simulink model "cascaded_with_phase_shifted"  (R2022b)
settings: Solver=ode3  StartTime=0.0  StopTime=0.5  FixedStep=5e-5  RelTol=1e-3
libraries: spsIGBTDiodeLib x8, simulink x4, spsDCVoltageSourceLib x2, spsVoltageMeasurementLib x1, sps_lib x1
settings Model: Creator=gudel  LastModifiedBy=gudel

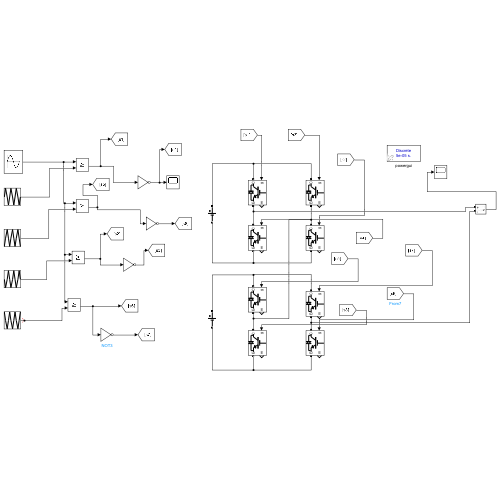
[thumbnail: Simulink's stored preview of the top-level diagram]
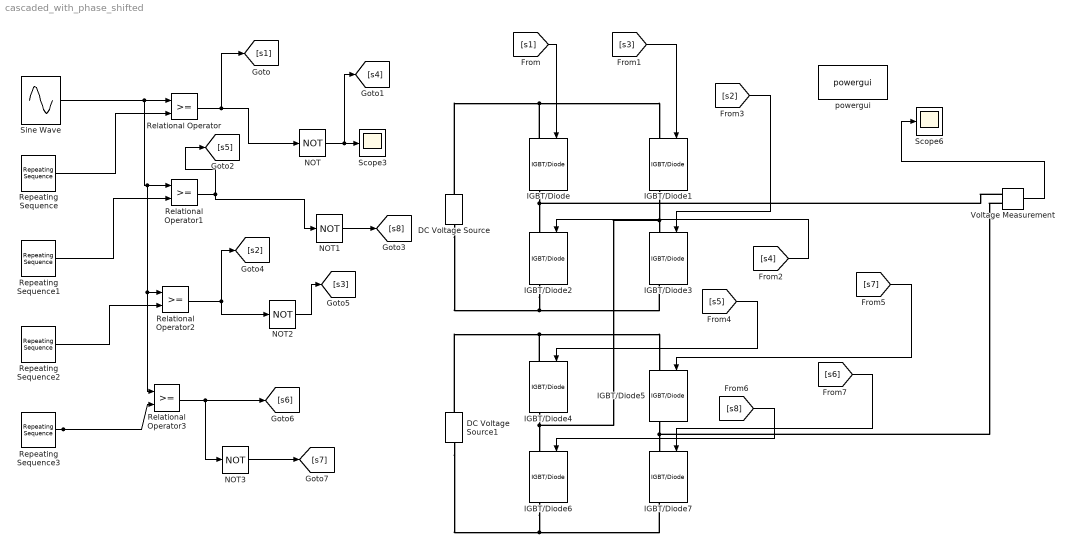
== system cascaded_with_phase_shifted ==
  DC Voltage Source : spsDCVoltageSourceLib/DC Voltage Source  Amplitude=100  Measurements=None
  DC Voltage Source1 : spsDCVoltageSourceLib/DC Voltage Source  Amplitude=100  Measurements=Voltage
  IGBT/Diode{,1..7} (8 alike) : spsIGBTDiodeLib/IGBT//Diode  Ron=1e-3  Rs=1e5  Cs=inf  Measurements=on
  NOT{,1..3} (4 alike) : Logic  Operator=NOT  IconShape=distinctive  AllPortsSameDT=off  OutDataTypeStr=boolean
  Relational Operator{,1..3} (4 alike) : RelationalOperator  OutDataTypeStr=boolean  RndMeth=Simplest  InputSameDT=off
  Repeating Sequence : simulink/Sources/Repeating Sequence  rep_seq_t=[0 0.25 0.5 0.75 1]*1/2000  rep_seq_y=[0 1 0 -1 0]
  Repeating Sequence1 : simulink/Sources/Repeating Sequence  rep_seq_t=[0 0.25 0.5 0.75 1]*1/2000  rep_seq_y=[-1 0 1 0 -1]
  Repeating Sequence2 : simulink/Sources/Repeating Sequence  rep_seq_t=[0 0.25 0.5 0.75 1]*1/2000  rep_seq_y=[0 -1 0 1 0]
  Repeating Sequence3 : simulink/Sources/Repeating Sequence  rep_seq_t=[0 0.25 0.5 0.75 1]*1/2000  rep_seq_y=[1 0 -1 0 1]
  Scope3 : Scope
  Scope6 : Scope
  Sine Wave : Sin  Frequency=2*pi*50  SampleTime=0
  Voltage Measurement : spsVoltageMeasurementLib/Voltage Measurement  PhasorSimulation=off  OutputType=Complex  PSBequivalent=0
  powergui : sps_lib/powergui  Priority=1  SimulationMode=Discrete  SampleTime=50e-6  frequency=60  Iterations=50  frequencyindice=0  Pbase=100e6  ErrMax=1e-4  UnitsV=kV  UnitsW=MW  buscounter=0  FunctionMessages=off  echomessages=off  EnableUseOfTLC=off  CurrentSourceSwitches=off  DisableSnubberDevices=off  DisableRonSwitches=off  DisableVfSwitches=off  DisplayEquations=off  AutomaticDiscreteSolvers=off  SolverType=Tustin/Backward Euler (TBE)  Interpol=off  ExternalGateDelay=off  methode=off  Ts=100  x0status=blocks  SPID=on  SwTol=0  HookPort=off  NonlinearTolerance=1e-4  nMaxIteration=100  ContinueOnMaxIteration=off  RestoreLinks=warning  ResistiveCurrentMeasurement=off  Frange=[0:2:500]  Ylog=off  Xlog=on  ShowGrid=off  save=off  variable=ZData  structure=0  ZoomFFT=off  StartTime=0.0  cycles=1  DisplayStyle=1  fundamental=60  FreqAxis=off  MaxFrequency=1000  frequencyindicesteady=1  RmsSteady=1  display=off
  wires:
  Sine Wave/1 -> Relational Operator3/1, Relational Operator2/1, Relational Operator1/1, Relational Operator/1
  Repeating Sequence/1 -> Relational Operator/2
  Repeating Sequence1/1 -> Relational Operator1/2
  Repeating Sequence2/1 -> Relational Operator2/2
  Relational Operator1/1 -> NOT1/1, [s5]
  Relational Operator2/1 -> [s2], NOT2/1
  NOT/1 -> [s4], Scope3/1
  NOT1/1 -> [s8]
  NOT2/1 -> [s3]
  [s1] -> IGBT/Diode/1
  [s3] -> IGBT/Diode1/1
  [s4] -> IGBT/Diode2/1
  [s2] -> IGBT/Diode3/1
  [s5] -> IGBT/Diode4/1
  [s7] -> IGBT/Diode5/1
  [s8] -> IGBT/Diode6/1
  [s6] -> IGBT/Diode7/1
  Relational Operator/1 -> [s1], NOT/1
  Repeating Sequence3/1 -> Relational Operator3/2
  Relational Operator3/1 -> NOT3/1, [s6]
  NOT3/1 -> [s7]
  Voltage Measurement/1 -> Scope6/1
  connections:
  IGBT/Diode/LConn1 -- IGBT/Diode1/LConn1 -- DC Voltage Source/RConn1
  IGBT/Diode2/RConn1 -- DC Voltage Source/LConn1 -- IGBT/Diode3/RConn1
  IGBT/Diode/RConn1 -- Voltage Measurement/LConn1 -- IGBT/Diode2/LConn1
  IGBT/Diode4/LConn1 -- DC Voltage Source1/RConn1 -- IGBT/Diode5/LConn1
  IGBT/Diode6/RConn1 -- DC Voltage Source1/LConn1 -- IGBT/Diode7/RConn1
  IGBT/Diode1/RConn1 -- IGBT/Diode6/LConn1 -- IGBT/Diode4/RConn1 -- IGBT/Diode3/LConn1
  IGBT/Diode5/RConn1 -- Voltage Measurement/LConn2 -- IGBT/Diode7/LConn1
